simulink model "balancingController_with_OOT_and_transfer"  (Simulink 8.4)
settings: Solver=FixedStepDiscrete  StartTime=0.0  StopTime=simulationTime  FixedStep=Ts  RelTol=1e-3
InitFcn:
  | initBalancingController_with_OOT_and_transfer;
values from neighbouring files (symbols this model uses):
  Ts = 0.01    [initBalancingController_with_OOT_and_transfer.m]
undefined symbols (not defined in the file or in its folder): CoMDes, CoMErrorThreshold, dampings, forceThreshold, gainMomentum, gainsDCOM, gainsICOM, gainsPCOM, impedances, NUMBER_OF_STATES, qDesCoM, qDesRightFoot, ROBOT_DOF_FOR_SIMULINK, smoothingTimeJacobians, tBalancing
undefined symbols (not defined in the file): localName, robotName
libraries: WBCLibrary x48
settings Model: Creator=daniele  LastModifiedBy=pucci
settings DataIOCC: SignalLoggingSaveFormat=Dataset
settings DebuggingCC: FcnCallInpInsideContextMsg=EnableAllAsWarning
settings SFSimCC: SimParseCustomCode=off

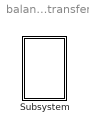
== system balancingController_with_OOT_and_transfer ==
  Subsystem : Subsystem  mask{robotName=robotName, Ts=Ts, localName=localName}
      mask prompts: robotName "robot name"; localName "module name"

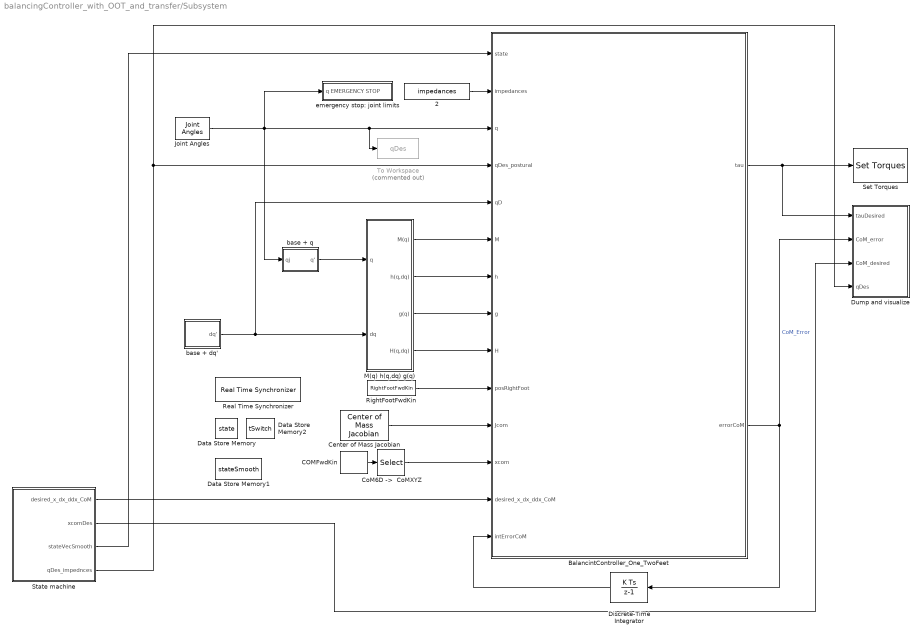
== system balancingController_with_OOT_and_transfer/Subsystem ==
  "    2" : Constant  Value=impedances
  BalancintController_One_TwoFeet : Subsystem
  "COMFwdKin " : WBCLibrary/wholeBodyModel/Forward Kinematics/COMFwdKin   robotName=robotName  localName=localName
  Center of Mass Jacobian : WBCLibrary/wholeBodyModel/Jacobians/Center of Mass Jacobian  robotName=robotName  localName=localName
  "CoM6D ->  CoMXYZ" : Selector  InputPortWidth=7  Indices=[1 2 3]
  Data Store Memory : DataStoreMemory  DataStoreName=state  OutDataTypeStr=double
  Data Store Memory1 : DataStoreMemory  DataStoreName=stateSmooth  InitialValue=[1,0,0,0]  OutDataTypeStr=double
  Data Store Memory2 : DataStoreMemory  DataStoreName=tSwitch  OutDataTypeStr=double
  Discrete-Time Integrator : DiscreteIntegrator  InitialCondition=[0 0 0]  SampleTime=Ts
  Dump and visualize : Subsystem
  Joint Angles : WBCLibrary/wholeBodyStates/Joint Angles  robotName=robotName  localName=localName
  M(q) h(q,dq) g(q) : Subsystem
  Real Time Synchronizer : WBCLibrary/Utilities/Real Time Synchronizer  Priority=-10  threadPeriod=Ts
  RightFootFwdKin : WBCLibrary/wholeBodyModel/Forward Kinematics/RightFootFwdKin  robotName=robotName  localName=localName
  Set Torques : WBCLibrary/wholeBodyActuators/Set Torques  val=6  robotName=robotName  localName=localName
  "State machine " : Subsystem
  To Workspace : ToWorkspace  Commented=on  VariableName=qDes  SaveFormat=Timeseries  SampleTime=-1
  base + dq' : Subsystem
  base + q : Subsystem
  emergency stop: joint limits : Subsystem
  wires:
  RightFootFwdKin/1 -> BalancintController_One_TwoFeet/10(posRightFoot)
  Discrete-Time Integrator/1 -> BalancintController_One_TwoFeet/14(intErrorCoM)
  base + q/1(q') -> M(q) h(q,dq) g(q)/1(q)
  M(q) h(q,dq) g(q)/3(g(q)) -> BalancintController_One_TwoFeet/8(g)
  M(q) h(q,dq) g(q)/4(H(q,dq)) -> BalancintController_One_TwoFeet/9(H)
  Center of Mass Jacobian/1 -> BalancintController_One_TwoFeet/11(Jcom)
  base + dq'/1(dq') -> BalancintController_One_TwoFeet/5(qD), M(q) h(q,dq) g(q)/2(dq)
  M(q) h(q,dq) g(q)/1(M(q)) -> BalancintController_One_TwoFeet/6(M)
  M(q) h(q,dq) g(q)/2(h(q,dq)) -> BalancintController_One_TwoFeet/7(h)
  BalancintController_One_TwoFeet/1(tau) -> Set Torques/1, Dump and visualize/1(tauDesired)
  Joint Angles/1 -> emergency stop: joint limits/1(q EMERGENCY STOP), To Workspace/1, BalancintController_One_TwoFeet/3(q), base + q/1(qj)
  BalancintController_One_TwoFeet/2(errorCoM) -> Discrete-Time Integrator/1, Dump and visualize/2(CoM_error)  "CoM_Error"
  "State machine "/2(xcomDes) -> Dump and visualize/3(CoM_desired)
  "COMFwdKin "/1 -> "CoM6D ->  CoMXYZ"/1
  "CoM6D ->  CoMXYZ"/1 -> BalancintController_One_TwoFeet/12(xcom)
  "State machine "/1(desired_x_dx_ddx_CoM) -> BalancintController_One_TwoFeet/13(desired_x_dx_ddx_CoM)
  "    2"/1 -> BalancintController_One_TwoFeet/2(impedances)
  "State machine "/3(stateVecSmooth) -> BalancintController_One_TwoFeet/1(state)
  "State machine "/4(qDes_impednces) -> Dump and visualize/4(qDes), BalancintController_One_TwoFeet/4(qDes_postural)

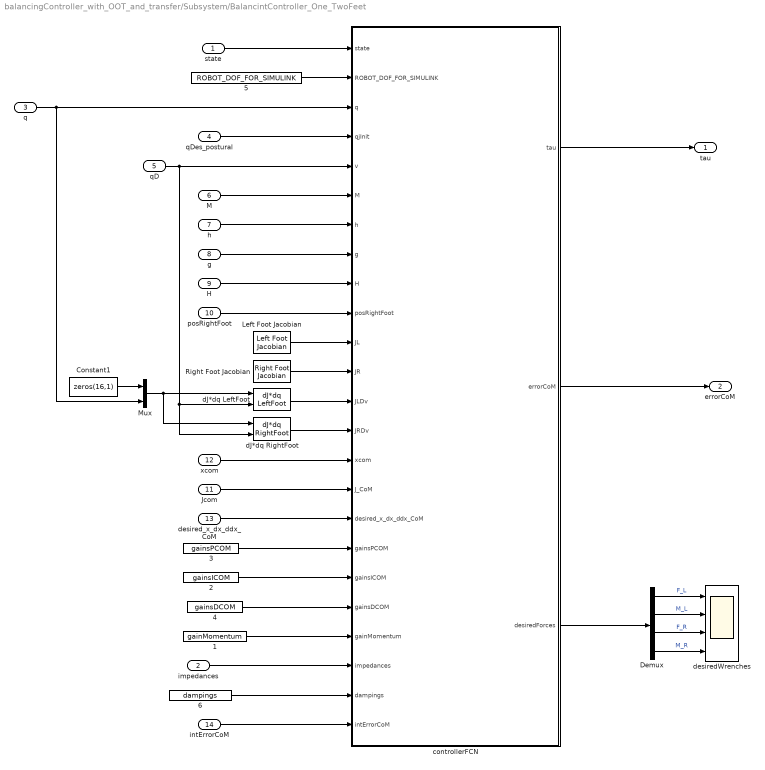
== system balancingController_with_OOT_and_transfer/Subsystem/BalancintController_One_TwoFeet ==
  state : Inport
  impedances : Inport  Port=2
  q : Inport  Port=3
  qDes_postural : Inport  Port=4
  qD : Inport  Port=5
  M : Inport  Port=6
  h : Inport  Port=7
  g : Inport  Port=8
  H : Inport  Port=9
  posRightFoot : Inport  Port=10
  Jcom : Inport  Port=11
  xcom : Inport  Port=12
  desired_x_dx_ddx_CoM : Inport  Port=13
  intErrorCoM : Inport  Port=14
  "    1" : Constant  Value=gainMomentum
  "    2" : Constant  Value=gainsICOM
  "    3" : Constant  Value=gainsPCOM
  "    4" : Constant  Value=gainsDCOM
  "    5" : Constant  Value=ROBOT_DOF_FOR_SIMULINK
  "    6" : Constant  Value=dampings
  Constant1 : Constant  Value=zeros(16,1)
  Demux : Demux
  Left Foot Jacobian : WBCLibrary/wholeBodyModel/Jacobians/Left Foot Jacobian  robotName=robotName  localName=localName
  Mux : Mux  Inputs=2
  Right Foot Jacobian : WBCLibrary/wholeBodyModel/Jacobians/Right Foot Jacobian  robotName=robotName  localName=localName
  controllerFCN : MATLAB Function  TreatAsAtomicUnit=on
  dJ*dq LeftFoot : WBCLibrary/wholeBodyModel/Dynamics/dJ*dq LeftFoot  val=9  robotName=robotName  localName=localName
  dJ*dq RightFoot : WBCLibrary/wholeBodyModel/Dynamics/dJ*dq RightFoot  val=9  robotName=robotName  localName=localName
  desiredWrenches : Scope  NumInputPorts=4
      settings: ShowLegends=on  TimeRange=150  YMin=-5~-5~63.70967741935465~-5  YMax=5~5~150~5  SaveName=ScopeData2
  tau : Outport
  errorCoM : Outport  Port=2
  wires:
  q/1 -> Mux/2, controllerFCN/3(q)
  qDes_postural/1 -> controllerFCN/4(qjInit)
  qD/1 -> dJ*dq RightFoot/2, dJ*dq LeftFoot/2, controllerFCN/5(v)
  M/1 -> controllerFCN/6(M)
  h/1 -> controllerFCN/7(h)
  g/1 -> controllerFCN/8(g)
  H/1 -> controllerFCN/9(H)
  posRightFoot/1 -> controllerFCN/10(posRightFoot)
  Left Foot Jacobian/1 -> controllerFCN/11(JL)
  Right Foot Jacobian/1 -> controllerFCN/12(JR)
  xcom/1 -> controllerFCN/15(xcom)
  Jcom/1 -> controllerFCN/16(J_CoM)
  desired_x_dx_ddx_CoM/1 -> controllerFCN/17(desired_x_dx_ddx_CoM)
  impedances/1 -> controllerFCN/22(impedances)
  intErrorCoM/1 -> controllerFCN/24(intErrorCoM)
  "    3"/1 -> controllerFCN/18(gainsPCOM)
  "    1"/1 -> controllerFCN/21(gainMomentum)
  "    2"/1 -> controllerFCN/19(gainsICOM)
  "    4"/1 -> controllerFCN/20(gainsDCOM)
  controllerFCN/1(tau) -> tau/1
  controllerFCN/2(errorCoM) -> errorCoM/1
  "    5"/1 -> controllerFCN/2(ROBOT_DOF_FOR_SIMULINK)
  "    6"/1 -> controllerFCN/23(dampings)
  controllerFCN/3(desiredForces) -> Demux/1
  Demux/1 -> desiredWrenches/1  "F_L"
  Demux/2 -> desiredWrenches/2  "M_L"
  Demux/3 -> desiredWrenches/3  "F_R"
  Demux/4 -> desiredWrenches/4  "M_R"
  state/1 -> controllerFCN/1(state)
  dJ*dq LeftFoot/1 -> controllerFCN/13(JLDv)
  dJ*dq RightFoot/1 -> controllerFCN/14(JRDv)
  Constant1/1 -> Mux/1
  Mux/1 -> dJ*dq RightFoot/1, dJ*dq LeftFoot/1

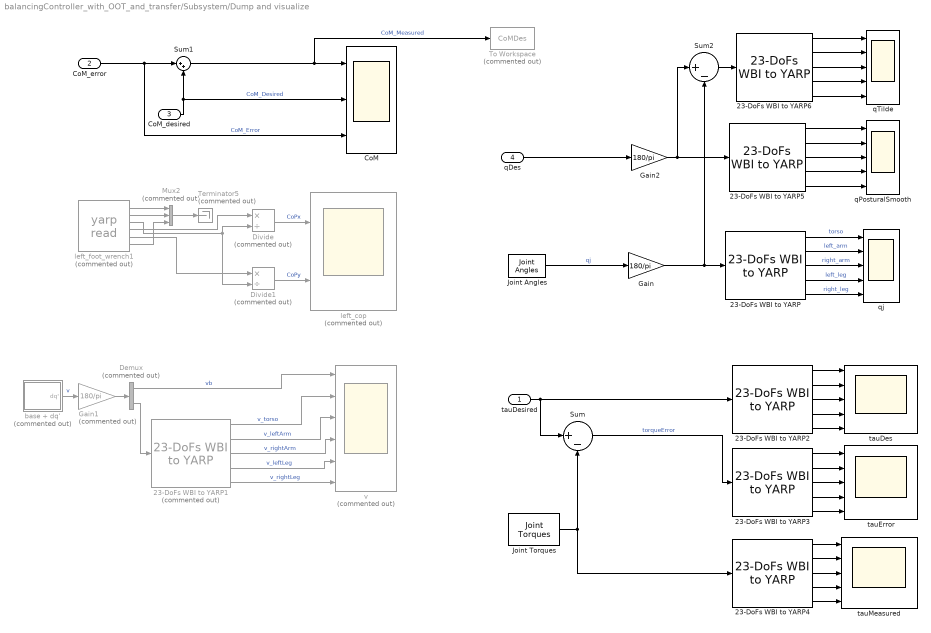
== system balancingController_with_OOT_and_transfer/Subsystem/Dump and visualize ==
  tauDesired : Inport
  CoM_error : Inport  Port=2
  CoM_desired : Inport  Port=3
  qDes : Inport  Port=4
  23-DoFs WBI to YARP{,2..6} (6 alike) : WBCLibrary/Utilities/23-DoFs WBI to YARP
  23-DoFs WBI to YARP1 : WBCLibrary/Utilities/23-DoFs WBI to YARP  Commented=on
  CoM : Scope  NumInputPorts=3
      settings: ShowLegends=on  TimeRange=400  YMin=-0.2~-0.2~-0.006  YMax=0.5~0.5~0.004  SaveName=CoM_data
  Demux : Demux  Commented=on  Outputs=2
  Divide : Product  Commented=on  Inputs=*/
  Divide1 : Product  Commented=on  Inputs=*/
  Gain : Gain  Gain=180/pi
  Gain1 : Gain  Commented=on  Gain=180/pi
  Gain2 : Gain  Gain=180/pi
  Joint Angles : WBCLibrary/wholeBodyStates/Joint Angles  robotName=robotName  localName=localName
  Joint Torques : WBCLibrary/wholeBodyStates/Joint Torques  robotName=robotName  localName=localName
  Mux2 : Mux  Commented=on  Inputs=3
  Sum : Sum  Inputs=|+-
  Sum1 : Sum  Inputs=|++
  Sum2 : Sum  Inputs=|+-
  Terminator5 : Terminator  Commented=on
  To Workspace : ToWorkspace  Commented=on  VariableName=CoMDes  SaveFormat=Timeseries  SampleTime=-1
  base + dq' : Subsystem  Commented=on
  left_cop : Scope  Commented=on  NumInputPorts=2
      settings: ShowLegends=on  TimeRange=42.68  YMin=-50~-20  YMax=250~180  SaveName=ScopeData6
  left_foot_wrench1 : WBCLibrary/Utilities/yarp read  Commented=on  from=['/wholeBodyDynamicsTree/filtered/l_foot_ft_sensor:o']  to='...'  num=6  blocking=off  timestamp=off  autoconnect=on
  qPosturalSmooth : Scope  NumInputPorts=5
      settings: ShowLegends=on  TimeRange=34.19  YMin=-0.4~-40~-40~-20~-20  YMax=0.4~60~60~20~20  SaveName=ScopeData3
  qTilde : Scope  NumInputPorts=5
      settings: ShowLegends=on  TimeRange=34.19  YMin=-0.4~-40~-40~-20~-20  YMax=0.4~60~60~20~20  SaveName=ScopeData5
  qj : Scope  NumInputPorts=5
      settings: ShowLegends=on  TimeRange=400  YMin=-40~-50~-50~-20~-40  YMax=20~100~100~40~40  SaveName=qj_and_v
  tauDes : Scope  NumInputPorts=5
      settings: ShowLegends=on  TimeRange=22.09  YMin=-30~-4~-10~-10~-10  YMax=10~4~5~10~10  SaveName=tauDes
  tauError : Scope  NumInputPorts=5
      settings: ShowLegends=on  TimeRange=18.63  YMin=-1~-1~-1.5~-10~-10  YMax=2~1~1~15~15  SaveName=tauError
  tauMeasured : Scope  NumInputPorts=5
      settings: ShowLegends=on  TimeRange=4.26  YMin=-5~-5~-2~-5~-5  YMax=5~5~2~5~5  SaveName=tauMeasured
  v : Scope  Commented=on  NumInputPorts=6
      settings: ShowLegends=on  TimeRange=10  YMin=-0.124~-5~-5~-5~-5~-5  YMax=-0.106~5~5~5~5~5  SaveName=qj_and_v1
  wires:
  CoM_error/1 -> CoM/3, Sum1/1  "CoM_Error"
  tauDesired/1 -> 23-DoFs WBI to YARP2/1, Sum/1
  23-DoFs WBI to YARP3/3 -> tauError/3
  23-DoFs WBI to YARP2/4 -> tauDes/4
  23-DoFs WBI to YARP3/4 -> tauError/4
  23-DoFs WBI to YARP2/3 -> tauDes/3
  23-DoFs WBI to YARP4/4 -> tauMeasured/4
  23-DoFs WBI to YARP3/1 -> tauError/1
  23-DoFs WBI to YARP4/5 -> tauMeasured/5
  Joint Torques/1 -> 23-DoFs WBI to YARP4/1, Sum/2
  23-DoFs WBI to YARP4/3 -> tauMeasured/3
  23-DoFs WBI to YARP4/2 -> tauMeasured/2
  CoM_desired/1 -> Sum1/2, CoM/2  "CoM_Desired"
  23-DoFs WBI to YARP3/2 -> tauError/2
  23-DoFs WBI to YARP4/1 -> tauMeasured/1
  Sum1/1 -> To Workspace/1, CoM/1  "CoM_Measured"
  23-DoFs WBI to YARP3/5 -> tauError/5
  23-DoFs WBI to YARP2/1 -> tauDes/1
  Sum/1 -> 23-DoFs WBI to YARP3/1  "torqueError"
  23-DoFs WBI to YARP2/2 -> tauDes/2
  23-DoFs WBI to YARP2/5 -> tauDes/5
  base + dq'/1(dq') -> Gain1/1  "v"
  Joint Angles/1 -> Gain/1  "qj"
  Gain/1 -> Sum2/2, 23-DoFs WBI to YARP/1
  23-DoFs WBI to YARP/5 -> qj/5  "right_leg"
  23-DoFs WBI to YARP/1 -> qj/1  "torso"
  23-DoFs WBI to YARP/2 -> qj/2  "left_arm"
  23-DoFs WBI to YARP/4 -> qj/4  "left_leg"
  23-DoFs WBI to YARP/3 -> qj/3  "right_arm"
  Gain1/1 -> Demux/1
  Demux/2 -> 23-DoFs WBI to YARP1/1
  23-DoFs WBI to YARP1/5 -> v/6  "v_rightLeg"
  23-DoFs WBI to YARP1/4 -> v/5  "v_leftLeg"
  23-DoFs WBI to YARP1/3 -> v/4  "v_rightArm"
  23-DoFs WBI to YARP1/2 -> v/3  "v_leftArm"
  23-DoFs WBI to YARP1/1 -> v/2  "v_torso"
  Demux/1 -> v/1  "vb"
  23-DoFs WBI to YARP5/3 -> qPosturalSmooth/3
  23-DoFs WBI to YARP5/1 -> qPosturalSmooth/1
  23-DoFs WBI to YARP5/2 -> qPosturalSmooth/2
  23-DoFs WBI to YARP5/4 -> qPosturalSmooth/4
  Gain2/1 -> Sum2/1, 23-DoFs WBI to YARP5/1
  qDes/1 -> Gain2/1
  23-DoFs WBI to YARP5/5 -> qPosturalSmooth/5
  23-DoFs WBI to YARP6/3 -> qTilde/3
  23-DoFs WBI to YARP6/1 -> qTilde/1
  23-DoFs WBI to YARP6/2 -> qTilde/2
  23-DoFs WBI to YARP6/4 -> qTilde/4
  23-DoFs WBI to YARP6/5 -> qTilde/5
  Sum2/1 -> 23-DoFs WBI to YARP6/1
  left_foot_wrench1/2 -> Mux2/2
  left_foot_wrench1/4 -> Divide/1
  left_foot_wrench1/5 -> Divide1/1
  left_foot_wrench1/6 -> Mux2/3
  left_foot_wrench1/3 -> Divide/2, Divide1/2
  left_foot_wrench1/1 -> Mux2/1
  Mux2/1 -> Terminator5/1
  Divide/1 -> left_cop/1  "CoPx"
  Divide1/1 -> left_cop/2  "CoPy"

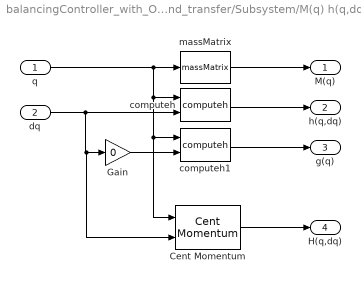
== system balancingController_with_OOT_and_transfer/Subsystem/M(q) h(q,dq) g(q) ==
  q : Inport
  dq : Inport  Port=2
  Cent Momentum : WBCLibrary/wholeBodyModel/Dynamics/Cent Momentum  robotName=robotName  localName=localName
  Gain : Gain  Gain=0
  computeh : WBCLibrary/wholeBodyModel/Dynamics/computeh  val=7  robotname=robotName  localname=localName
  computeh1 : WBCLibrary/wholeBodyModel/Dynamics/computeh  val=7  robotname=robotName  localname=localName
  massMatrix : WBCLibrary/wholeBodyModel/Dynamics/massMatrix  val=8  robotname=robotName  localname=localName
  M(q) : Outport
  h(q,dq) : Outport  Port=2
  g(q) : Outport  Port=3
  H(q,dq) : Outport  Port=4
  wires:
  Gain/1 -> computeh1/2
  computeh1/1 -> g(q)/1
  computeh/1 -> h(q,dq)/1
  massMatrix/1 -> M(q)/1
  q/1 -> Cent Momentum/1, computeh1/1, computeh/1, massMatrix/1
  dq/1 -> Cent Momentum/2, Gain/1, computeh/2
  Cent Momentum/1 -> H(q,dq)/1

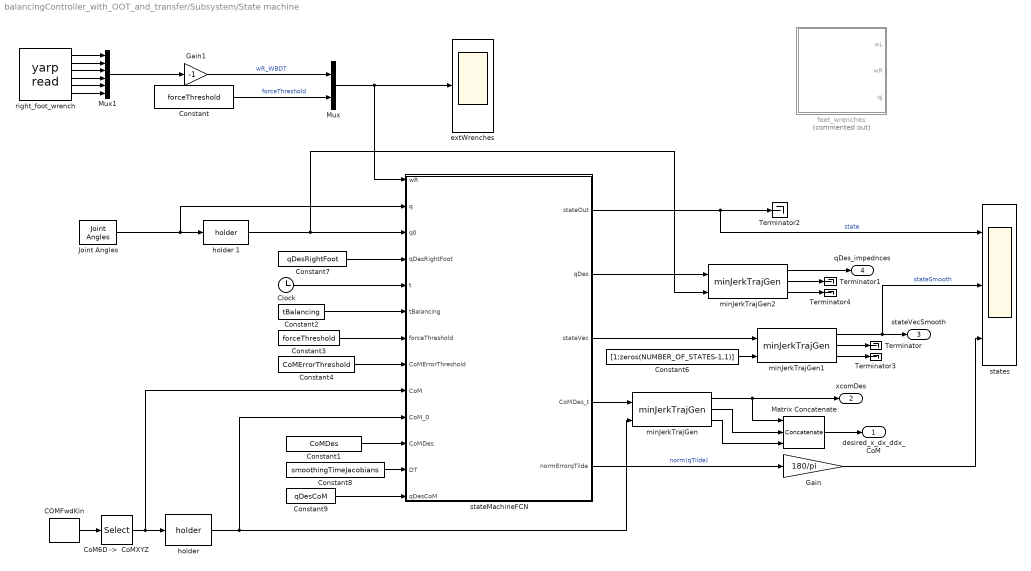
== system balancingController_with_OOT_and_transfer/Subsystem/State machine  ==
  "COMFwdKin " : WBCLibrary/wholeBodyModel/Forward Kinematics/COMFwdKin   robotName=robotName  localName=localName
  Clock : Clock
  "CoM6D ->  CoMXYZ" : Selector  InputPortWidth=7  Indices=[1 2 3]
  Constant : Constant  Value=forceThreshold
  Constant1 : Constant  Value=CoMDes
  Constant2 : Constant  Value=tBalancing
  Constant3 : Constant  Value=forceThreshold
  Constant4 : Constant  Value=CoMErrorThreshold
  Constant6 : Constant  Value=[1;zeros(NUMBER_OF_STATES-1,1)]
  Constant7 : Constant  Value=qDesRightFoot
  Constant8 : Constant  Value=smoothingTimeJacobians
  Constant9 : Constant  Value=qDesCoM
  Gain : Gain  Gain=180/pi
  Gain1 : Gain  Gain=-1
  Joint Angles : WBCLibrary/wholeBodyStates/Joint Angles  robotName=robotName  localName=localName
  Matrix Concatenate : Concatenate  NumInputs=3  Mode=Multidimensional array  ConcatenateDimension=2
  Mux : Mux  Inputs=2
  Mux1 : Mux  Inputs=6
  Terminator{,1..4} (5 alike) : Terminator
  extWrenches : Scope
      settings: ShowLegends=on  TimeRange=42.68  YMin=-50  YMax=250
  feet_wrenches : Subsystem  Commented=on
  "holder " : WBCLibrary/Utilities/holder 
  holder 1 : WBCLibrary/Utilities/holder 
  minJerkTrajGen : WBCLibrary/Utilities/minJerkTrajGen  dim=3  Ts=Ts  Tt=transferTime
  minJerkTrajGen1 : WBCLibrary/Utilities/minJerkTrajGen  dim=NUMBER_OF_STATES  Ts=Ts  Tt=smoothingTimeJacobians
  minJerkTrajGen2 : WBCLibrary/Utilities/minJerkTrajGen  dim=ROBOT_DOF  Ts=Ts  Tt=trajectoryTimePostural
  right_foot_wrench : WBCLibrary/Utilities/yarp read  from=['/wholeBodyDynamicsTree/filtered/r_foot_ft_sensor:o']  to=['...']  num=6  blocking=off  timestamp=off  autoconnect=on
  stateMachineFCN : MATLAB Function  TreatAsAtomicUnit=on
  states : Scope  NumInputPorts=3
      settings: ShowLegends=on  TimeRange=17.36  YMin=0~-0~0  YMax=4~1.2~30  SaveName=ScopeData4
  desired_x_dx_ddx_CoM : Outport
  xcomDes : Outport  Port=2
  stateVecSmooth : Outport  Port=3
  qDes_impednces : Outport  Port=4
  wires:
  "COMFwdKin "/1 -> "CoM6D ->  CoMXYZ"/1
  "CoM6D ->  CoMXYZ"/1 -> stateMachineFCN/9(CoM), "holder "/1
  minJerkTrajGen/1 -> Matrix Concatenate/1, xcomDes/1
  minJerkTrajGen/2 -> Matrix Concatenate/2
  minJerkTrajGen/3 -> Matrix Concatenate/3
  Matrix Concatenate/1 -> desired_x_dx_ddx_CoM/1
  Clock/1 -> stateMachineFCN/5(t)
  Constant2/1 -> stateMachineFCN/6(tBalancing)
  Constant3/1 -> stateMachineFCN/7(forceThreshold)
  Constant4/1 -> stateMachineFCN/8(CoMErrorThreshold)
  Constant1/1 -> stateMachineFCN/11(CoMDes)
  stateMachineFCN/1(stateOut) -> states/1, Terminator2/1  "state"
  "holder "/1 -> minJerkTrajGen/2, stateMachineFCN/10(CoM_0)
  Constant6/1 -> minJerkTrajGen1/2
  stateMachineFCN/3(stateVec) -> minJerkTrajGen1/1
  minJerkTrajGen1/1 -> stateVecSmooth/1, states/2  "stateSmooth"
  minJerkTrajGen1/2 -> Terminator/1
  holder 1/1 -> minJerkTrajGen2/2, stateMachineFCN/3(q0)
  stateMachineFCN/2(qDes) -> minJerkTrajGen2/1
  minJerkTrajGen2/1 -> qDes_impednces/1
  minJerkTrajGen1/3 -> Terminator3/1
  minJerkTrajGen2/2 -> Terminator1/1
  minJerkTrajGen2/3 -> Terminator4/1
  Mux/1 -> stateMachineFCN/1(wR), extWrenches/1
  Constant/1 -> Mux/2  "forceThreshold"
  Constant7/1 -> stateMachineFCN/4(qDesRightFoot)
  Constant8/1 -> stateMachineFCN/12(DT)
  Constant9/1 -> stateMachineFCN/13(qDesCoM)
  right_foot_wrench/2 -> Mux1/2
  right_foot_wrench/1 -> Mux1/1
  right_foot_wrench/4 -> Mux1/4
  right_foot_wrench/5 -> Mux1/5
  right_foot_wrench/6 -> Mux1/6
  right_foot_wrench/3 -> Mux1/3
  Mux1/1 -> Gain1/1
  stateMachineFCN/5(normErrorqTilde) -> Gain/1  "norm(qTilde)"
  Gain/1 -> states/3
  Joint Angles/1 -> stateMachineFCN/2(q), holder 1/1
  Gain1/1 -> Mux/1  "wR_WBDT"
  stateMachineFCN/4(CoMDes_t) -> minJerkTrajGen/1

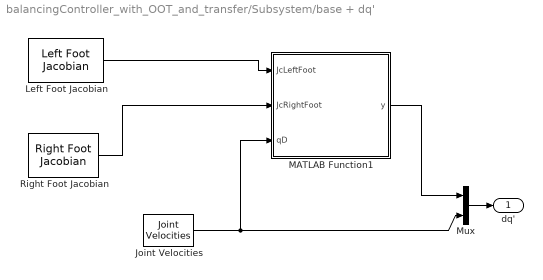
== system balancingController_with_OOT_and_transfer/Subsystem/base + dq' ==
  Joint Velocities : WBCLibrary/wholeBodyStates/Joint Velocities  robotName=robotName  localName=localName
  Left Foot Jacobian : WBCLibrary/wholeBodyModel/Jacobians/Left Foot Jacobian  robotName=robotName  localName=localName
  MATLAB Function1 : MATLAB Function  TreatAsAtomicUnit=on
  Mux : Mux  Inputs=2
  Right Foot Jacobian : WBCLibrary/wholeBodyModel/Jacobians/Right Foot Jacobian  robotName=robotName  localName=localName
  dq' : Outport
  wires:
  Left Foot Jacobian/1 -> MATLAB Function1/1(JcLeftFoot)
  MATLAB Function1/1(y) -> Mux/1
  Mux/1 -> dq'/1
  Right Foot Jacobian/1 -> MATLAB Function1/2(JcRightFoot)
  Joint Velocities/1 -> MATLAB Function1/3(qD), Mux/2

== system balancingController_with_OOT_and_transfer/Subsystem/base + q ==
  qj : Inport
  Constant1 : Constant  Value=zeros(16,1)
  Mux : Mux  Inputs=2
  q' : Outport
  wires:
  Mux/1 -> q'/1
  qj/1 -> Mux/2
  Constant1/1 -> Mux/1

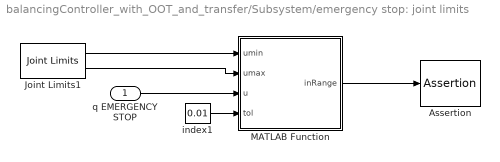
== system balancingController_with_OOT_and_transfer/Subsystem/emergency stop: joint limits ==
  q EMERGENCY STOP : Inport
  Assertion : Assertion
  Joint Limits1 : WBCLibrary/wholeBodyModel/Joint Limits  robotName=robotName  localName=localName
  MATLAB Function : MATLAB Function  TreatAsAtomicUnit=on
  index1 : Constant  Value=0.01  VectorParams1D=off
  wires:
  Joint Limits1/1 -> MATLAB Function/1(umin)
  Joint Limits1/2 -> MATLAB Function/2(umax)
  index1/1 -> MATLAB Function/4(tol)
  q EMERGENCY STOP/1 -> MATLAB Function/3(u)
  MATLAB Function/1(inRange) -> Assertion/1

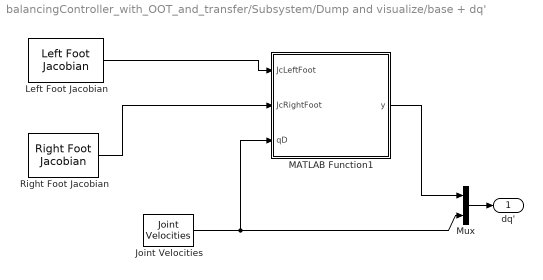
== system balancingController_with_OOT_and_transfer/Subsystem/Dump and visualize/base + dq' ==
  Joint Velocities : WBCLibrary/wholeBodyStates/Joint Velocities  robotName=robotName  localName=localName
  Left Foot Jacobian : WBCLibrary/wholeBodyModel/Jacobians/Left Foot Jacobian  robotName=robotName  localName=localName
  MATLAB Function1 : MATLAB Function  TreatAsAtomicUnit=on
  Mux : Mux  Inputs=2
  Right Foot Jacobian : WBCLibrary/wholeBodyModel/Jacobians/Right Foot Jacobian  robotName=robotName  localName=localName
  dq' : Outport
  wires:
  Left Foot Jacobian/1 -> MATLAB Function1/1(JcLeftFoot)
  MATLAB Function1/1(y) -> Mux/1
  Mux/1 -> dq'/1
  Right Foot Jacobian/1 -> MATLAB Function1/2(JcRightFoot)
  Joint Velocities/1 -> MATLAB Function1/3(qD), Mux/2

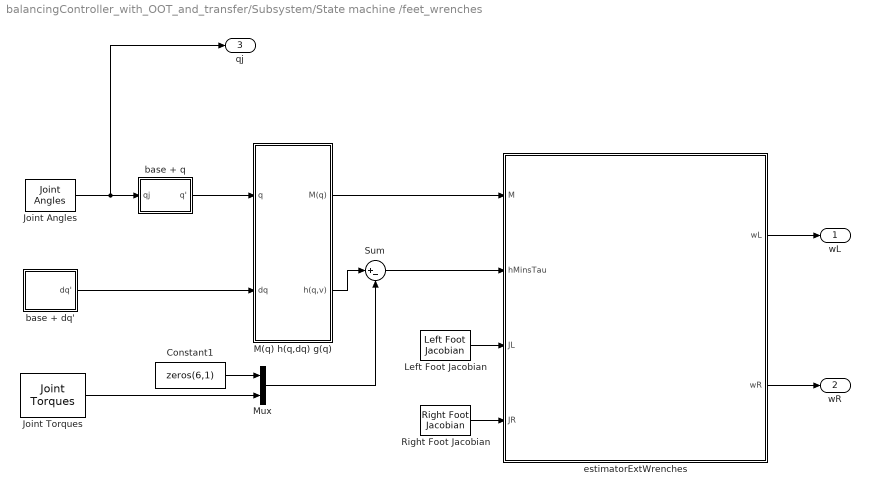
== system balancingController_with_OOT_and_transfer/Subsystem/State machine /feet_wrenches ==
  Constant1 : Constant  Value=zeros(6,1)
  Joint Angles : WBCLibrary/wholeBodyStates/Joint Angles  robotName=robotName  localName=localName
  Joint Torques : WBCLibrary/wholeBodyStates/Joint Torques  robotName=robotName  localName=localName
  Left Foot Jacobian : WBCLibrary/wholeBodyModel/Jacobians/Left Foot Jacobian  robotName=robotName  localName=localName
  M(q) h(q,dq) g(q) : Subsystem
  Mux : Mux  Inputs=2
  Right Foot Jacobian : WBCLibrary/wholeBodyModel/Jacobians/Right Foot Jacobian  robotName=robotName  localName=localName
  Sum : Sum  Inputs=|+-
  base + dq' : Subsystem
  base + q : Subsystem
  estimatorExtWrenches : MATLAB Function  TreatAsAtomicUnit=on
  wL : Outport
  wR : Outport  Port=2
  qj : Outport  Port=3
  wires:
  Right Foot Jacobian/1 -> estimatorExtWrenches/4(JR)
  base + q/1(q') -> M(q) h(q,dq) g(q)/1(q)
  Left Foot Jacobian/1 -> estimatorExtWrenches/3(JL)
  estimatorExtWrenches/2(wR) -> wR/1
  base + dq'/1(dq') -> M(q) h(q,dq) g(q)/2(dq)
  M(q) h(q,dq) g(q)/1(M(q)) -> estimatorExtWrenches/1(M)
  Joint Angles/1 -> qj/1, base + q/1(qj)
  estimatorExtWrenches/1(wL) -> wL/1
  M(q) h(q,dq) g(q)/2(h(q,v)) -> Sum/1
  Sum/1 -> estimatorExtWrenches/2(hMinsTau)
  Mux/1 -> Sum/2
  Constant1/1 -> Mux/1
  Joint Torques/1 -> Mux/2

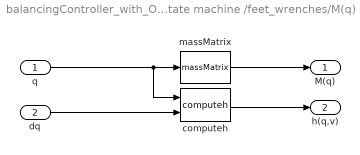
== system balancingController_with_OOT_and_transfer/Subsystem/State machine /feet_wrenches/M(q) h(q,dq) g(q) ==
  q : Inport
  dq : Inport  Port=2
  computeh : WBCLibrary/wholeBodyModel/Dynamics/computeh  val=7  robotname=robotName  localname=localName
  massMatrix : WBCLibrary/wholeBodyModel/Dynamics/massMatrix  val=8  robotname=robotName  localname=localName
  M(q) : Outport
  h(q,v) : Outport  Port=2
  wires:
  computeh/1 -> h(q,v)/1
  massMatrix/1 -> M(q)/1
  q/1 -> computeh/1, massMatrix/1
  dq/1 -> computeh/2

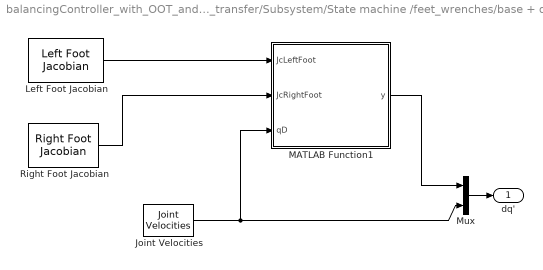
== system balancingController_with_OOT_and_transfer/Subsystem/State machine /feet_wrenches/base + dq' ==
  Joint Velocities : WBCLibrary/wholeBodyStates/Joint Velocities  robotName=robotName  localName=localName
  Left Foot Jacobian : WBCLibrary/wholeBodyModel/Jacobians/Left Foot Jacobian  robotName=robotName  localName=localName
  MATLAB Function1 : MATLAB Function  TreatAsAtomicUnit=on
  Mux : Mux  Inputs=2
  Right Foot Jacobian : WBCLibrary/wholeBodyModel/Jacobians/Right Foot Jacobian  robotName=robotName  localName=localName
  dq' : Outport
  wires:
  Left Foot Jacobian/1 -> MATLAB Function1/1(JcLeftFoot)
  MATLAB Function1/1(y) -> Mux/1
  Mux/1 -> dq'/1
  Right Foot Jacobian/1 -> MATLAB Function1/2(JcRightFoot)
  Joint Velocities/1 -> MATLAB Function1/3(qD), Mux/2

== system balancingController_with_OOT_and_transfer/Subsystem/State machine /feet_wrenches/base + q ==
  qj : Inport
  Constant1 : Constant  Value=zeros(16,1)
  Mux : Mux  Inputs=2
  q' : Outport
  wires:
  Mux/1 -> q'/1
  qj/1 -> Mux/2
  Constant1/1 -> Mux/1

== matlab function Subsystem/State machine /stateMachineFCN ==
  data: stateOut output double; qDes output double; stateVec output double; CoMDes_t output double; state data_store_memory double; wR input double; q input double; q0 input double; qDesRightFoot input double; t input double; tBalancing input double; forceThreshold input double; CoMErrorThreshold input double; CoM input double; CoM_0 input double; CoMDes input double; tSwitch data_store_memory double; DT input double; qDesCoM input double; normErrorqTilde output double
function [stateOut,qDes,stateVec,CoMDes_t,normErrorqTilde]  = stateMachineFCN(wR,q,q0,qDesRightFoot,t,tBalancing,forceThreshold,CoMErrorThreshold,CoM,CoM_0,CoMDes,DT,qDesCoM)
%#codegen
global state;
global tSwitch;

normErrorqTilde = 0;
CoMDes_t     = CoM_0;
stateVec   = zeros(4,1);
qDes       = q0;
if state == 0 
    stateVec = [1;0;0;0];
    if t > tBalancing
       state = 1; 
    end
end
if state == 1 
    stateVec = [0;1;0;0];
    CoMDes_t(2) =  CoMDes(1,2);
    CoMError  = CoMDes_t - CoM;
    qDes = qDesCoM;
    if  norm(CoMError) < CoMErrorThreshold %%wR(3) < forceThreshold &&
       state = 2; 
       tSwitch = t;
    end
end

if state == 2 
    stateVec = [0;0;1;0];
    CoMDes_t(2) =  CoMDes(1,2);
    qDes = qDesCoM;
    if t > tSwitch + DT
        qDes(end-11:end)      =  qDesRightFoot(1,end-11:end);
        normErrorqTilde = norm(qDes(end-11:end) - q(end-11:end));
        if  normErrorqTilde < 7.5*pi/180
            state = 3; 
        end
    end
end

if state == 3
    stateVec = [0;0;1;0];
    qDes(end-11:end)      =  qDesRightFoot(2,end-11:end);
    CoMDes_t     = CoMDes(2,:)';
%     CoMError  = CoMDes_t - CoM;
    if  abs(wR(3)) > forceThreshold  %norm(CoMError) < CoMErrorThreshold && 
       state = 4; 
       tSwitch = t;
    end
end

if state == 4
  	stateVec = [1;0;0;0];
    qDes(end-11:end)      =  qDesRightFoot(2,end-11:end);
    CoMDes_t     = CoMDes(2,:)';
end

stateOut = state;

== matlab function Subsystem/base + dq'/MATLAB Function1 ==
  data: JcLeftFoot input double; JcRightFoot input double; y output double; qD input double; stateSmooth data_store_memory double
function y = fcn(JcLeftFoot,JcRightFoot,qD)
%#codegen
global stateSmooth;

Jc = [JcLeftFoot;JcRightFoot*(1-stateSmooth(3))];

y = -pinv(Jc(:,1:6))*Jc(:,7:end)*qD;

== matlab function Subsystem/BalancintController_One_TwoFeet/controllerFCN ==
  data: state input double; ROBOT_DOF_FOR_SIMULINK input double; q input double; tau output double; qjInit input double; v input double; M input double; h input double; g input double; H input double; posRightFoot input double; JL input double; JR input double; JLDv input double; JRDv input double; xcom input double; J_CoM input double; desired_x_dx_ddx_CoM input double; gainsPCOM input double; gainsICOM input double; gainsDCOM input double; gainMomentum input double; impedances input double; dampings input double; intErrorCoM input double; errorCoM output double; desiredForces output double
function [tau,errorCoM,desiredForces]   =  controllerFCN(state,ROBOT_DOF_FOR_SIMULINK,q,qjInit,v, M, h, g, H, posRightFoot, JL,JR, JLDv,JRDv, xcom,J_CoM, desired_x_dx_ddx_CoM, gainsPCOM,gainsICOM,gainsDCOM,gainMomentum, impedances,dampings, intErrorCoM)
%#codegen

desiredForces   = zeros(12,1);
ROBOT_DOF       = size(ROBOT_DOF_FOR_SIMULINK,1);
PINV_TOL        = 1e-5;
reg             = 0.01;
gravAcc         = 9.81;
m               = M(1,1);
Mb              = M(1:6,1:6);
Mbj             = M(1:6,7:end);
% Mj              = M(7:end,7:end);

St              = [  zeros(6,ROBOT_DOF);
                   eye(ROBOT_DOF,ROBOT_DOF)];
grav            = [ zeros(2,1);
                   -m*gravAcc;
                    zeros(3,1)];
pos_rightFoot   = posRightFoot(1:3);

xDcom           = J_CoM(1:3,:)*v;
qD              = v(7:end);
xDDcomStar      = desired_x_dx_ddx_CoM(:,3) - gainsPCOM*(xcom - desired_x_dx_ddx_CoM(:,1)) - gainsICOM*intErrorCoM - gainsDCOM*(xDcom - desired_x_dx_ddx_CoM(:,2));
Pr              = pos_rightFoot - xcom; % Application point of the contact force on the right foot w.r.t. CoM


AL = [ eye(3),   zeros(3);
      -Sf(xcom),  eye(3)];
AR = [ eye(3), zeros(3);
        Sf(Pr), eye(3) ];
    
A    = [ AL, AR];

Jc   = [ JL ;
         JR*(1-state(3))];
JcDv = [ JLDv ;
         JRDv*(1-state(3))];

JcMinv          = Jc/M;
JcMinvSt        = JcMinv*St;
JcMinvJct       = JcMinv*transpose(Jc);

pinvA         = pinv( A, PINV_TOL)*(1-state(3)) + [inv(AL);zeros(6)]*state(3); 
% PInv_JcMinvSt = pinv( JcMinvSt, PINV_TOL);
PInv_JcMinvSt = JcMinvSt'/(JcMinvSt*JcMinvSt' + reg*eye(size(JcMinvSt,1)));
  
HDotDes  = [ m*xDDcomStar ;
            -gainMomentum*H(4:end)]; 
         
%% QP FOR TORQUE MINIMIZATION BASED ON arbitrary vector F0
% Maux = [     eye(3)     zeros(3,22)
%           zeros(22,3)      inv(Mj(4:end,4:end))];
%define tau_0 (the arbitrary vector)
N0_tau        = eye(ROBOT_DOF) - PInv_JcMinvSt*JcMinvSt;

mult_f_tau0   =  Mbj'/Mb*transpose(Jc(:,1:6))-transpose(Jc(:,7:end)); % multiplier of f in tau0
n_tau0        =  h(7:end) - Mbj'/Mb*h(1:6) - diag(impedances)*(q-qjInit)  -diag(dampings)*N0_tau*qD ; % additional terms in tau0 - Mj*(kPandD_Postural(1,:)'.*(q-qjInit) + kPandD_Postural(2,:)'.*qD) 
%

mult_f_tau    = -PInv_JcMinvSt*JcMinvJct    + N0_tau*mult_f_tau0;

% f desired is given as:
% f*   = pinvA*(HDotDes - grav)  + (I-pinvA*A) * f0
% f*   =           f_HDot        +     N0_f    * f0
f_HDot = pinvA*(HDotDes - grav);

% tau is given as:
% tau = (mult_f_tau*N0_f)* f0 + (n_tau+mult_f_tau*f_HDot)
% tau =        X_tau     * f0 +                   Y_tau

Y_tau            = PInv_JcMinvSt*(JcMinv*h-JcDv) + N0_tau*n_tau0 + mult_f_tau*f_HDot;

N0_f             =  eye(12,12)-pinvA*A;
X_tau            = mult_f_tau*N0_f;
f0               = -pinv(X_tau)*Y_tau;
tau              = X_tau   * f0*(1-state(3))   +  Y_tau;
desiredForces    = N0_f    * f0*(1-state(3))   +  f_HDot;

errorCoM = xcom - desired_x_dx_ddx_CoM(:,1);

== matlab function Subsystem/emergency stop: joint limits/MATLAB Function ==
  data: umin input double; umax input double; u input double; inRange output double; tol input double
function inRange = checkRange(umin, umax, u, tol)
%#codegen

res = u < umin + tol | u > umax - tol;
res = sum(res);
if res==0
    inRange = 1;
else
    inRange = 0;
    u < umin + tol | u > umax - tol
end

== matlab function Subsystem/Dump and visualize/base + dq'/MATLAB Function1 ==
  data: JcLeftFoot input double; JcRightFoot input double; y output double; qD input double; stateSmooth data_store_memory double
function y = fcn(JcLeftFoot,JcRightFoot,qD)
%#codegen
global stateSmooth;

Jc = [JcLeftFoot;JcRightFoot*(1-stateSmooth(3))];

y = -pinv(Jc(:,1:6))*Jc(:,7:end)*qD;

== matlab function Subsystem/State machine /feet_wrenches/base + dq'/MATLAB Function1 ==
  data: JcLeftFoot input double; JcRightFoot input double; y output double; qD input double; stateSmooth data_store_memory double
function y = fcn(JcLeftFoot,JcRightFoot,qD)
%#codegen
global stateSmooth;

Jc = [JcLeftFoot;JcRightFoot*(1-stateSmooth(3))];

y = -pinv(Jc(:,1:6))*Jc(:,7:end)*qD;

== matlab function Subsystem/State machine /feet_wrenches/estimatorExtWrenches ==
  data: wL output double; state data_store_memory double; M input double; hMinsTau input double; JL input double; JR input double; wR output double
function [wL,wR]  = stateMachineFCN(M,hMinsTau,JL,JR)
%#codegen
    global state;
    wL = zeros(6,1);
    wR = zeros(6,1);
    if state == 0 || state == 1 || state == 2
       J  = [JL;JR];
       f  = (J/M*J')\(J/M)*hMinsTau;
       wL = f(1:6);
       wR = f(7:end);
    end
    
%     if state == 2
%        J  = [JL];
%        f  = (J/M*J')\(J/M)*hMinsTau;
%        wL = f(1:6);
%     end

end
